simulink model "simplificado"  (R2023a)
settings: Solver=VariableStepAuto  StartTime=0.0  StopTime=400  RelTol=1e-3
values from neighbouring files (symbols this model uses):
  A1 = 0.0154    [parametros.m]    (also in variables.mat)
  A2 = 5e-5    (= 5e-05)    [parametros.m]    (also in variables.mat)
  az = 0.5    [parametros.m]    (also in variables.mat)
  g = 9.8    [parametros.m]    (also in variables.mat)
  H_ini = 0    [parametros.m]    (also in variables.mat)
  H_star = H_max/2    (= 0.31)    [parametros.m]    (also in variables.mat)
  ro = 1000    [parametros.m]    (also in variables.mat)
libraries: rllib x1
settings Model: Creator=emmanuel  LastModifiedBy=empg0
settings OptimizationCC: ReuseModelBlockBuffer=off

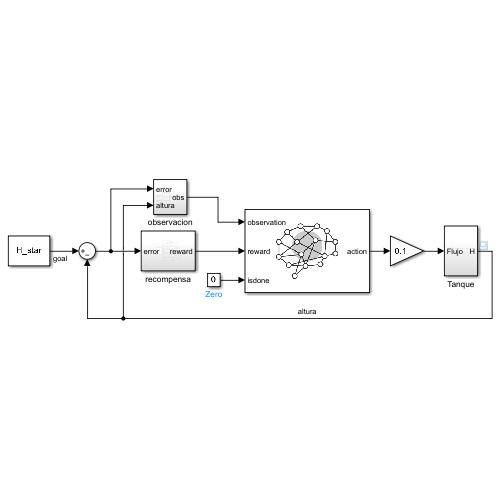
[thumbnail: Simulink's stored preview of the top-level diagram]
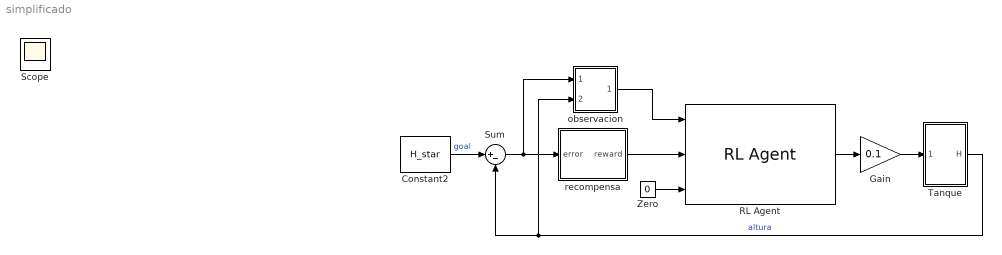
== system simplificado ==
  Constant2 : Constant  Value=H_star
  Gain : Gain  Gain=0.1
  RL Agent : rllib/RL Agent  Agent=agent  ExternalActionAsInput=off  ProvideLastAction=off  ProvideCumRwd=off  TreatAsDirectFeedthrough=on  UseStrictObservationDataTypes=off
  Sum : Sum  Inputs=|+-
  Tanque : Subsystem
  Zero : Constant  Value=0  OutDataTypeStr=Inherit: Inherit via back propagation
  observacion : Subsystem
  recompensa : Subsystem
  Scope : Scope
  wires:
  Tanque/1(H) -> Sum/2, observacion/2(altura)  "altura"
  Sum/1 -> observacion/1(error), recompensa/1(error)
  observacion/1(obs) -> RL Agent/1
  Constant2/1 -> Sum/1  "goal"
  recompensa/1(reward) -> RL Agent/2
  RL Agent/1 -> Gain/1
  Gain/1 -> Tanque/1(Flujo)
  Zero/1 -> RL Agent/3

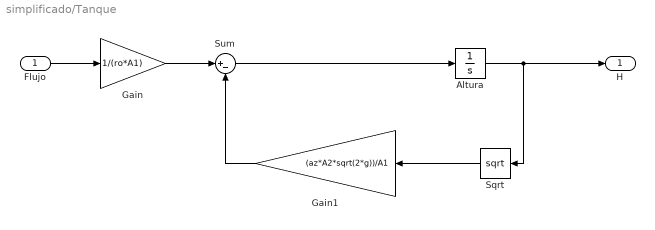
== system simplificado/Tanque ==
  Flujo : Inport
  Altura : Integrator  InitialCondition=H_ini  LimitOutput=on  UpperSaturationLimit=0.62  LowerSaturationLimit=0
  Gain : Gain  Gain=1/(ro*A1)
  Gain1 : Gain  Gain=(az*A2*sqrt(2*g))/A1
  Sqrt : Sqrt
  Sum : Sum  Inputs=|+-
  H : Outport
  wires:
  Gain/1 -> Sum/1
  Sum/1 -> Altura/1
  Sqrt/1 -> Gain1/1
  Gain1/1 -> Sum/2
  Altura/1 -> H/1, Sqrt/1
  Flujo/1 -> Gain/1

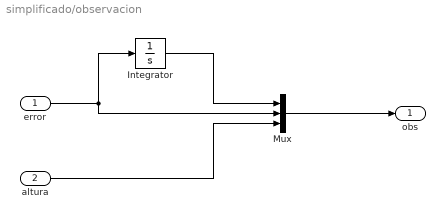
== system simplificado/observacion ==
  error : Inport
  altura : Inport  Port=2
  Integrator : Integrator
  Mux : Mux  Inputs=3
  obs : Outport
  wires:
  Integrator/1 -> Mux/1
  error/1 -> Integrator/1, Mux/2
  Mux/1 -> obs/1
  altura/1 -> Mux/3

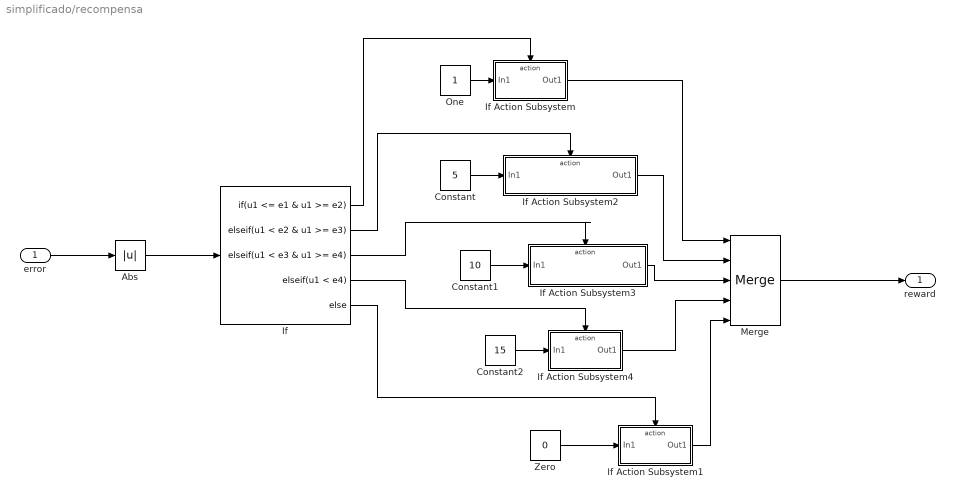
== system simplificado/recompensa ==
  error : Inport
  Abs : Abs  SaturateOnIntegerOverflow=off
  Constant : Constant  Value=5
  Constant1 : Constant  Value=10
  Constant2 : Constant  Value=15
  If : If  IfExpression=u1 <= e1 & u1 >= e2  ElseIfExpressions=u1 < e2 & u1 >= e3, u1 < e3 & u1 >= e4, u1 < e4
  If Action Subsystem : Subsystem  TreatAsAtomicUnit=on
  If Action Subsystem1 : Subsystem  TreatAsAtomicUnit=on
  If Action Subsystem2 : Subsystem  TreatAsAtomicUnit=on
  If Action Subsystem3 : Subsystem  TreatAsAtomicUnit=on
  If Action Subsystem4 : Subsystem  TreatAsAtomicUnit=on
  Merge : Merge  Inputs=5
  One : Constant  OutDataTypeStr=Inherit: Inherit via back propagation
  Zero : Constant  Value=0  OutDataTypeStr=Inherit: Inherit via back propagation
  reward : Outport
  wires:
  Abs/1 -> If/1
  error/1 -> Abs/1
  If/1 -> If Action Subsystem/Action
  Zero/1 -> If Action Subsystem1/1(In1)
  One/1 -> If Action Subsystem/1(In1)
  Merge/1 -> reward/1
  If/2 -> If Action Subsystem2/Action
  Constant/1 -> If Action Subsystem2/1(In1)
  If/3 -> If Action Subsystem3/Action
  Constant1/1 -> If Action Subsystem3/1(In1)
  If/4 -> If Action Subsystem4/Action
  If/5 -> If Action Subsystem1/Action
  Constant2/1 -> If Action Subsystem4/1(In1)
  If Action Subsystem/1(Out1) -> Merge/1
  If Action Subsystem2/1(Out1) -> Merge/2
  If Action Subsystem3/1(Out1) -> Merge/3
  If Action Subsystem4/1(Out1) -> Merge/4
  If Action Subsystem1/1(Out1) -> Merge/5

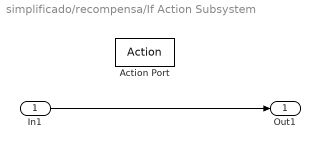
== system simplificado/recompensa/If Action Subsystem ==
  In1 : Inport
  Action Port : ActionPort  ActionPortLabel=if(u1 <= e1 & u1 >= e2)
  Out1 : Outport
  wires:
  In1/1 -> Out1/1

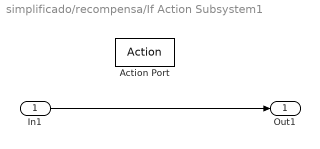
== system simplificado/recompensa/If Action Subsystem1 ==
  In1 : Inport
  Action Port : ActionPort  ActionPortLabel=else
  Out1 : Outport
  wires:
  In1/1 -> Out1/1

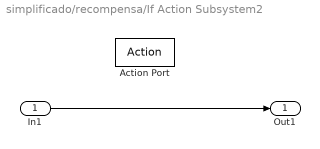
== system simplificado/recompensa/If Action Subsystem2 ==
  In1 : Inport
  Action Port : ActionPort  ActionPortLabel=elseif(u1 < e2 & u1 >= e3)
  Out1 : Outport
  wires:
  In1/1 -> Out1/1

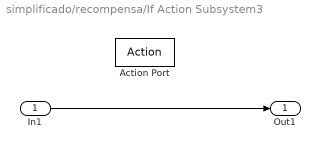
== system simplificado/recompensa/If Action Subsystem3 ==
  In1 : Inport
  Action Port : ActionPort  ActionPortLabel=elseif( u1 < e3 & u1 >= e4)
  Out1 : Outport
  wires:
  In1/1 -> Out1/1

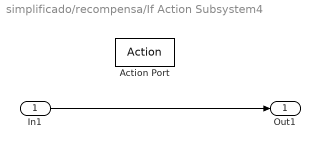
== system simplificado/recompensa/If Action Subsystem4 ==
  In1 : Inport
  Action Port : ActionPort  ActionPortLabel=elseif( u1 < e4)
  Out1 : Outport
  wires:
  In1/1 -> Out1/1
